simulink model "LRMate200Experimentor_Robot"  (R2015b)
settings: Solver=FixedStepDiscrete  StartTime=0.0  StopTime=10.0  FixedStep=si.SolverTimeStep  RelTol=1e-3
model workspace (MATLAB code in the model file):
  | rsi = evalin('base', 'si.ri{1}');
undefined symbols (not defined in the file or in its folder): si
libraries: simulink x4
(part 1 of 2)
settings Model: xpc_rtwmakecfg_data=_xpcethercatlib_  ParameterArgumentNames=rsi  Creator=rluser  LastModifiedBy=Te Tang
settings SolverCC: EnableConcurrentExecution=on
settings DataIOCC: SaveFormat=Array
settings OptimizationCC: BlockReduction=off  OptimizeBlockIOStorage=off  BufferReuse=off  GlobalBufferReuse=off  ExpressionFolding=off  LocalBlockOutputs=off
settings DebuggingCC: SolverPrmCheckMsg=warning  MultiTaskDSMMsg=none
settings HardwareCC: ProdBitPerPointer=32  ProdLargestAtomicFloat=None  ProdWordSize=32  ProdLongLongMode=on  ProdHWDeviceType=Generic->32-bit x86 compatible
settings RTWCC: SystemTargetFile=slrt.tlc  TemplateMakefile=slrt_default_tmf  Description=Simulink Real-Time  RTWCompilerOptimization=on
settings CodeAppCC: MaxIdLength=120
settings SimulinkRealTimeCC: GeneratePreprocessorConditionals=Disable all
settings ConfigComp: CovModelRefEnable=Off  CovSFcnEnable=off

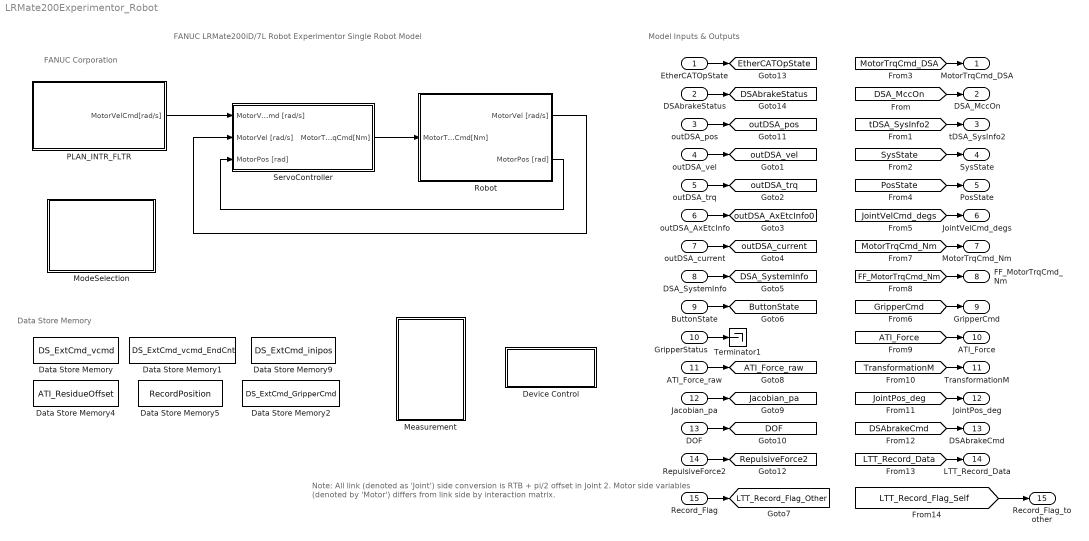
== system LRMate200Experimentor_Robot ==
  note: Model Inputs & Outputs
  note: Data Store Memory
  note: FANUC LRMate200iD/7L Robot Experimentor
      | Single Robot Model
  note: FANUC Corporation
  note: Note: All link (denoted as 'Joint') side conversion is RTB + pi/2 offset in Joint 2.
      | Motor side variables (denoted by 'Motor') differs from link side by interaction matrix.
  EtherCATOpState : Inport
  DSAbrakeStatus : Inport  Port=2
  outDSA_pos : Inport  Port=3
  outDSA_vel : Inport  Port=4
  outDSA_trq : Inport  Port=5
  outDSA_AxEtcInfo : Inport  Port=6
  outDSA_current : Inport  Port=7
  DSA_SystemInfo : Inport  Port=8
  ButtonState : Inport  Port=9  OutDataTypeStr=Bus: ButtonState
  GripperStatus : Inport  Port=10  OutDataTypeStr=Bus: GripperStatus
  ATI_Force_raw : Inport  Port=11  PortDimensions=6
  Jacobian_pa : Inport  Port=12  PortDimensions=[6 6]
  DOF : Inport  Port=13
  RepulsiveForce2 : Inport  Port=14  PortDimensions=3
  Record_Flag : Inport  Port=15  OutDataTypeStr=boolean  PortDimensions=1
  Data Store Memory : DataStoreMemory  DataStoreName=DS_ExtCmd_vcmd  WriteAfterWriteMsg=warning  WriteAfterReadMsg=warning  InitialValue=zeros(si.ext_vel_max_cnt,si.AxisNum)  OutDataTypeStr=double
  Data Store Memory1 : DataStoreMemory  DataStoreName=DS_ExtCmd_vcmd_EndCnt  WriteAfterWriteMsg=warning  WriteAfterReadMsg=warning  OutDataTypeStr=double
  Data Store Memory2 : DataStoreMemory  DataStoreName=DS_ExtCmd_GripperCmd  WriteAfterWriteMsg=warning  WriteAfterReadMsg=warning  InitialValue=zeros(si.ext_vel_max_cnt,6)  OutDataTypeStr=double
  Data Store Memory4 : DataStoreMemory  DataStoreName=ATI_ResidueOffset  WriteAfterWriteMsg=warning  WriteAfterReadMsg=warning  InitialValue=zeros(6,1)  OutDataTypeStr=double
  Data Store Memory5 : DataStoreMemory  DataStoreName=RecordPosition  WriteAfterWriteMsg=warning  WriteAfterReadMsg=warning  InitialValue=zeros(6,1)  OutDataTypeStr=double
  Data Store Memory9 : DataStoreMemory  DataStoreName=DS_ExtCmd_inipos  WriteAfterWriteMsg=warning  WriteAfterReadMsg=warning  InitialValue=zeros(1,si.AxisNum)  VectorParams1D=off  OutDataTypeStr=double
  Device Control : Subsystem
  Measurement : Subsystem
  ModeSelection : Subsystem
  PLAN_INTR_FLTR : Subsystem
  Robot : Subsystem
  ServoController : Subsystem  SystemSampleTime=si.tsv
  Terminator1 : Terminator
  MotorTrqCmd_DSA : Outport
  DSA_MccOn : Outport  Port=2
  tDSA_SysInfo2 : Outport  Port=3
  SysState : Outport  Port=4  OutDataTypeStr=Bus: SysState
  PosState : Outport  Port=5  OutDataTypeStr=Bus: PosState
  JointVelCmd_degs : Outport  Port=6
  MotorTrqCmd_Nm : Outport  Port=7
  FF_MotorTrqCmd_Nm : Outport  Port=8
  GripperCmd : Outport  Port=9  OutDataTypeStr=Bus: GripperCmd
  ATI_Force : Outport  Port=10
  TransformationM : Outport  Port=11
  JointPos_deg : Outport  Port=12
  DSAbrakeCmd : Outport  Port=13
  LTT_Record_Data : Outport  Port=14
  Record_Flag_to other : Outport  Port=15  OutDataTypeStr=boolean  PortDimensions=1
  tag scope: ATI_Force_raw=global, ButtonState=global, DOF=global, DSA_SystemInfo=global, DSAbrakeStatus=global, EtherCATOpState=global, Jacobian_pa=global, LTT_Record_Flag_Other=global, RepulsiveForce2=global, outDSA_AxEtcInfo0=global, outDSA_current=global, outDSA_pos=global, outDSA_trq=global, outDSA_vel=global
  wires:
  PLAN_INTR_FLTR/1(MotorVelCmd[rad/s]) -> ServoController/1(MotorVelCmd [rad/s])
  ServoController/1(MotorTrqCmd[Nm]) -> Robot/1(MotorTrqCmd[Nm])
  Robot/2(MotorPos [rad]) -> ServoController/3(MotorPos [rad])
  Robot/1(MotorVel [rad/s]) -> ServoController/2(MotorVel [rad/s])
  [MotorTrqCmd_DSA] -> MotorTrqCmd_DSA/1
  [DSA_MccOn] -> DSA_MccOn/1
  [tDSA_SysInfo2] -> tDSA_SysInfo2/1
  outDSA_pos/1 -> [outDSA_pos]
  outDSA_vel/1 -> [outDSA_vel]
  outDSA_trq/1 -> [outDSA_trq]
  outDSA_AxEtcInfo/1 -> [outDSA_AxEtcInfo0]
  outDSA_current/1 -> [outDSA_current]
  DSA_SystemInfo/1 -> [DSA_SystemInfo]
  ButtonState/1 -> [ButtonState]
  GripperStatus/1 -> Terminator1/1
  [SysState] -> SysState/1
  [PosState] -> PosState/1
  [JointVelCmd_degs] -> JointVelCmd_degs/1
  [MotorTrqCmd_Nm] -> MotorTrqCmd_Nm/1
  [FF_MotorTrqCmd_Nm] -> FF_MotorTrqCmd_Nm/1
  [GripperCmd] -> GripperCmd/1
  [ATI_Force] -> ATI_Force/1
  [TransformationM] -> TransformationM/1
  ATI_Force_raw/1 -> [ATI_Force_raw]
  [JointPos_deg] -> JointPos_deg/1
  Jacobian_pa/1 -> [Jacobian_pa]
  DOF/1 -> [DOF]
  RepulsiveForce2/1 -> [RepulsiveForce2]
  EtherCATOpState/1 -> [EtherCATOpState]
  DSAbrakeStatus/1 -> [DSAbrakeStatus]
  [DSAbrakeCmd] -> DSAbrakeCmd/1
  [LTT_Record_Data] -> LTT_Record_Data/1
  Record_Flag/1 -> [LTT_Record_Flag_Other]
  [LTT_Record_Flag_Self] -> Record_Flag_to other/1

== system LRMate200Experimentor_Robot/Device Control ==
  Gripper Input : Subsystem
  tag scope: GripperCmd=global
  wires:
  Gripper Input/1(GripperInput) -> [GripperCmd]

== system LRMate200Experimentor_Robot/Measurement ==
  Force Sensor : Subsystem
  LTT Handle : Subsystem
  Position State : Subsystem
  System State : Subsystem
  Terminator1 : Terminator
  Terminator4 : Terminator
  Terminator5 : Terminator
  Tilt Angle Esimation : Subsystem
  tag scope: ATI_Force=global, Green_ButtonE=global, LTT_ButtonE=global, LTT_Force=global, LTT_Record_Data=global, PosState=global, SysState=global, TCP_Force=global
  wires:
  System State/1(System State) -> [SysState]
  Position State/1(Position State) -> [PosState]
  Force Sensor/1(ATI_Force) -> [ATI_Force]
  Force Sensor/2(TCP_Force) -> [TCP_Force]
  LTT Handle/1(Green_Button) -> [Green_ButtonE]
  LTT Handle/2(RecordData) -> [LTT_Record_Data]
  LTT Handle/3(LTT_ButtonEnable) -> [LTT_ButtonE]
  Tilt Angle Esimation/1(Panel_RecordData) -> Terminator5/1
  Tilt Angle Esimation/2(TiltANA_col) -> Terminator4/1
  Tilt Angle Esimation/3(Estimated Tilt Angle) -> Terminator1/1
  Force Sensor/3(LTT_Force) -> [LTT_Force]

== system LRMate200Experimentor_Robot/ModeSelection ==
  Basic Control Mode : Subsystem
  LTT : Subsystem
  Pos Run & Jog : Subsystem

== system LRMate200Experimentor_Robot/PLAN_INTR_FLTR ==
  Basic : Subsystem
  JOG C : Subsystem
  LTT : Subsystem
  Peg Hole Insertion : Subsystem
  MotorVelCmd[rad/s] : Outport
  wires:
  Basic/1(MotorVelCmd[rad/s]) -> MotorVelCmd[rad/s]/1

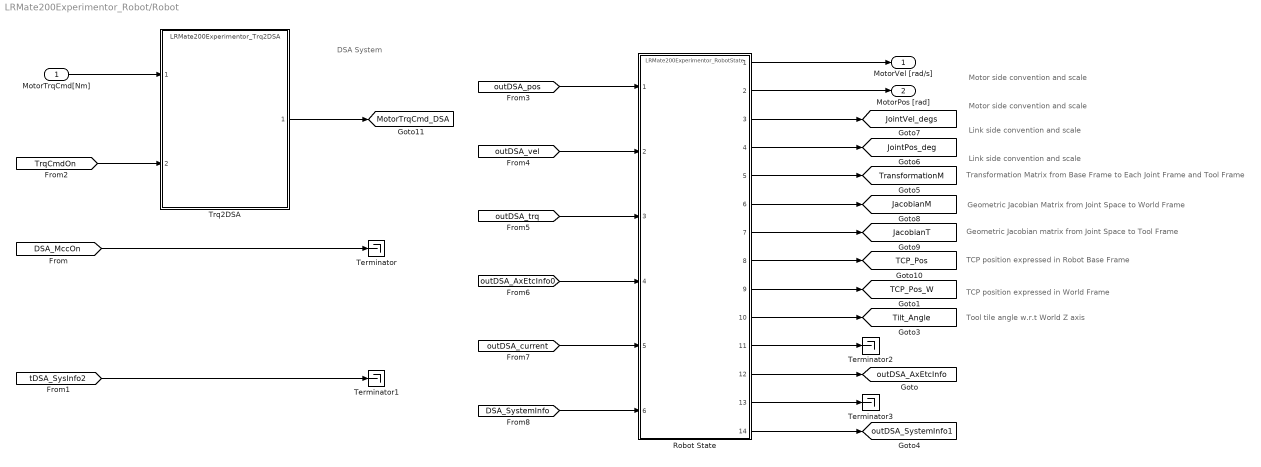
== system LRMate200Experimentor_Robot/Robot ==
  note: Motor side convention and scale
  note: TCP position expressed in Robot Base Frame
  note: Geometric Jacobian matrix from Joint Space to Tool Frame
  note: Geometric Jacobian Matrix from Joint Space to World Frame
  note: Transformation Matrix from Base Frame to Each Joint Frame and Tool Frame
  note: DSA System
  note: Motor side convention and scale
  note: Link side convention and scale
  note: Link side convention and scale
  note: Tool tile angle w.r.t World Z axis
  note: TCP position expressed in World Frame
  MotorTrqCmd[Nm] : Inport
  Robot State : ModelReference  ModelNameDialog=LRMate200Experimentor_RobotState.slx  ParameterArgumentNames=rsi  ParameterArgumentValues=rsi  SimulationMode=Normal  ModelReferenceVersion=1.185  CopyOfModelName=LRMate200Experimentor_RobotState.slx
  Terminator{,1..3} (4 alike) : Terminator
  Trq2DSA : ModelReference  ModelNameDialog=LRMate200Experimentor_Trq2DSA.slx  ParameterArgumentNames=rsi  ParameterArgumentValues=rsi  SimulationMode=Normal  ModelReferenceVersion=1.89  CopyOfModelName=LRMate200Experimentor_Trq2DSA.slx
  MotorVel [rad/s] : Outport
  MotorPos [rad] : Outport  Port=2
  tag scope: JacobianM=global, JacobianT=global, JointPos_deg=global, JointVel_degs=global, MotorTrqCmd_DSA=global, TCP_Pos=global, TCP_Pos_W=global, Tilt_Angle=global, TransformationM=global, outDSA_AxEtcInfo=global, outDSA_SystemInfo1=global
  wires:
  MotorTrqCmd[Nm]/1 -> Trq2DSA/1
  [TrqCmdOn] -> Trq2DSA/2
  [DSA_MccOn] -> Terminator/1
  [tDSA_SysInfo2] -> Terminator1/1
  Robot State/1 -> MotorVel [rad/s]/1
  Robot State/2 -> MotorPos [rad]/1
  Robot State/3 -> [JointVel_degs]
  Robot State/4 -> [JointPos_deg]
  Robot State/5 -> [TransformationM]
  Robot State/6 -> [JacobianM]
  Robot State/7 -> [JacobianT]
  Robot State/8 -> [TCP_Pos]
  Trq2DSA/1 -> [MotorTrqCmd_DSA]
  [outDSA_pos] -> Robot State/1
  [outDSA_vel] -> Robot State/2
  [outDSA_trq] -> Robot State/3
  [outDSA_AxEtcInfo0] -> Robot State/4
  [outDSA_current] -> Robot State/5
  [DSA_SystemInfo] -> Robot State/6
  Robot State/10 -> [Tilt_Angle]
  Robot State/11 -> Terminator2/1
  Robot State/12 -> [outDSA_AxEtcInfo]
  Robot State/13 -> Terminator3/1
  Robot State/14 -> [outDSA_SystemInfo1]
  Robot State/9 -> [TCP_Pos_W]

== system LRMate200Experimentor_Robot/ServoController ==
  MotorVelCmd [rad/s] : Inport
  MotorVel [rad/s] : Inport  Port=2
  MotorPos [rad] : Inport  Port=3
  Servo Model : ModelReference  ModelNameDialog=LRMate200Experimentor_Servo.slx  ParameterArgumentNames=rsi  ParameterArgumentValues=rsi  SimulationMode=Normal  ModelReferenceVersion=1.76  CopyOfModelName=LRMate200Experimentor_Servo.slx
  MotorTrqCmd[Nm] : Outport
  tag scope: FF_MotorTrqCmd_Nm=global, MotorTrqCmd_Nm=global
  wires:
  MotorVelCmd [rad/s]/1 -> Servo Model/1
  MotorPos [rad]/1 -> Servo Model/3
  MotorVel [rad/s]/1 -> Servo Model/2
  [ZReset] -> Servo Model/4
  Servo Model/1 -> [MotorTrqCmd_Nm], MotorTrqCmd[Nm]/1
  Servo Model/2 -> [FF_MotorTrqCmd_Nm]

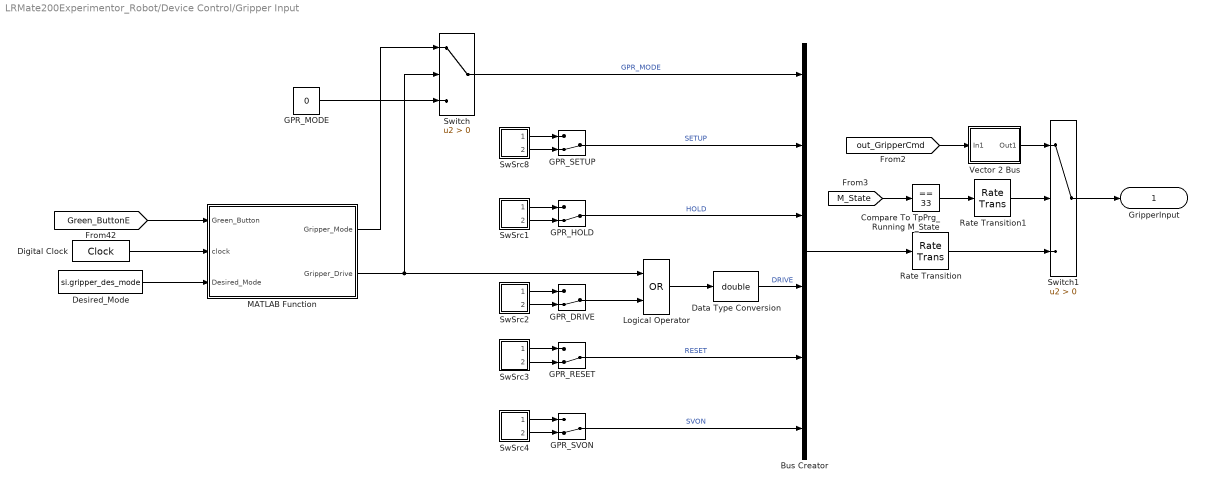
== system LRMate200Experimentor_Robot/Device Control/Gripper Input ==
  Bus Creator : BusCreator  Inputs=6
  Compare To TpPrg_Running M_State : simulink/Logic and Bit Operations/Compare To Constant  relop===  const=33  OutDataTypeStr=boolean
  Data Type Conversion : DataTypeConversion  OutDataTypeStr=double
  Desired_Mode : Constant  Value=si.gripper_des_mode
  Digital Clock : DigitalClock  SampleTime=0.001
  GPR_DRIVE : ManualSwitch  CurrentSetting=0
  GPR_HOLD : ManualSwitch  CurrentSetting=0
  GPR_MODE : Constant  Value=0
  GPR_RESET : ManualSwitch  CurrentSetting=0
  GPR_SETUP : ManualSwitch  CurrentSetting=0
  GPR_SVON : ManualSwitch  CurrentSetting=0
  Logical Operator : Logic  Operator=OR  AllPortsSameDT=off  OutDataTypeStr=boolean
  MATLAB Function : MATLAB Function  TreatAsAtomicUnit=on
  Rate Transition : RateTransition  OutPortSampleTime=si.timeGripperInputHold
  Rate Transition1 : RateTransition  OutPortSampleTime=si.timeGripperInputHold
  SwSrc1 : Subsystem
  SwSrc2 : Subsystem
  SwSrc3 : Subsystem
  SwSrc4 : Subsystem
  SwSrc8 : Subsystem
  Switch : Switch  Criteria=u2 > Threshold
  Switch1 : Switch  Criteria=u2 > Threshold
  Vector 2 Bus : Subsystem
  GripperInput : Outport
  wires:
  GPR_SVON/1 -> Bus Creator/6  "SVON"
  SwSrc8/2(ST0) -> GPR_SETUP/2
  SwSrc1/2(ST0) -> GPR_HOLD/2
  SwSrc4/2(ST0) -> GPR_SVON/2
  SwSrc1/1(ST1) -> GPR_HOLD/1
  SwSrc8/1(ST1) -> GPR_SETUP/1
  GPR_HOLD/1 -> Bus Creator/3  "HOLD"
  GPR_SETUP/1 -> Bus Creator/2  "SETUP"
  GPR_RESET/1 -> Bus Creator/5  "RESET"
  SwSrc2/2(ST0) -> GPR_DRIVE/2
  SwSrc3/2(ST0) -> GPR_RESET/2
  SwSrc4/1(ST1) -> GPR_SVON/1
  SwSrc3/1(ST1) -> GPR_RESET/1
  SwSrc2/1(ST1) -> GPR_DRIVE/1
  Digital Clock/1 -> MATLAB Function/2(clock)
  [Green_ButtonE] -> MATLAB Function/1(Green_Button)
  Logical Operator/1 -> Data Type Conversion/1
  GPR_DRIVE/1 -> Logical Operator/2
  MATLAB Function/2(Gripper_Drive) -> Switch/2, Logical Operator/1
  Switch/1 -> Bus Creator/1  "GPR_MODE"
  GPR_MODE/1 -> Switch/3
  MATLAB Function/1(Gripper_Mode) -> Switch/1
  Data Type Conversion/1 -> Bus Creator/4  "DRIVE"
  [out_GripperCmd] -> Vector 2 Bus/1(In1)
  Compare To TpPrg_Running M_State/1 -> Rate Transition1/1
  Bus Creator/1 -> Rate Transition/1
  Vector 2 Bus/1(Out1) -> Switch1/1
  Switch1/1 -> GripperInput/1
  Rate Transition/1 -> Switch1/3
  Rate Transition1/1 -> Switch1/2
  [M_State] -> Compare To TpPrg_Running M_State/1
  Desired_Mode/1 -> MATLAB Function/3(Desired_Mode)

== system LRMate200Experimentor_Robot/Measurement/Force Sensor ==
  ATI_Offset : Constant  Value=rsi.ATI_Offset
  Calibratioin Matrix : Gain  Gain=rsi.CalibrationMatrix  Multiplication=Matrix(K*u) (u vector)
  Data Store Read : DataStoreRead  DialogController=Simulink.DDGSource  DataStoreName=ATI_ResidueOffset  SampleTime=si.tsv
  Discrete Filter : DiscreteFilter  Numerator=si.Filter.num  Denominator=si.Filter.den  SampleTime=si.tsv
  Discrete Filter1 : DiscreteFilter  Numerator=si.Filter.num  Denominator=si.Filter.den  SampleTime=si.tsv
  Gravity Compensator : MATLAB Function  TreatAsAtomicUnit=on
  L_ATI2LTT : Constant  Value=rsi.L_ATI2LTT
  L_ATI2TCP : Constant  Value=rsi.L_ATI2TCP
  MATLAB Function6 : MATLAB Function  TreatAsAtomicUnit=on
  PayloadCG : Constant  Value=rsi.PayloadCG
  PayloadG : Constant  Value=rsi.PayloadG
  Substract : Sum  Inputs=+---
  ATI_Force : Outport
  TCP_Force : Outport  Port=2
  LTT_Force : Outport  Port=3
  wires:
  PayloadCG/1 -> Gravity Compensator/3(PayloadCG)
  [ATI_Force_raw] -> Calibratioin Matrix/1
  [TransformationM] -> Gravity Compensator/1(T)
  PayloadG/1 -> Gravity Compensator/2(PayloadG)
  Gravity Compensator/1(W) -> Discrete Filter1/1
  ATI_Offset/1 -> Substract/2
  Discrete Filter1/1 -> Substract/3
  Substract/1 -> ATI_Force/1, MATLAB Function6/1(ATI_Force)
  Calibratioin Matrix/1 -> Discrete Filter/1
  Discrete Filter/1 -> Substract/1
  Data Store Read/1 -> Substract/4
  MATLAB Function6/1(TCP_Force) -> TCP_Force/1
  L_ATI2TCP/1 -> MATLAB Function6/2(L_ATI2TCP)
  L_ATI2LTT/1 -> MATLAB Function6/3(L_ATI2LTT)
  MATLAB Function6/2(LTT_Force) -> LTT_Force/1

== system LRMate200Experimentor_Robot/Measurement/LTT Handle ==
  Bus Selector : BusSelector  OutputSignals=Green_Button,LTT_Button
  Digital Clock : DigitalClock  SampleTime=0.001
  LTT_RecordData_On : Constant  Value=0
  MATLAB Function : MATLAB Function  TreatAsAtomicUnit=on
  Mux : Mux  Inputs=3
  Rate Transition : RateTransition
  Rate Transition1 : RateTransition
  Green_Button : Outport
  RecordData : Outport  Port=2
  LTT_ButtonEnable : Outport  Port=3
  tag scope: LTT_Record_Flag_Self=global
  wires:
  MATLAB Function/1(RecordData) -> RecordData/1
  Digital Clock/1 -> MATLAB Function/4(clock)
  MATLAB Function/2(LTT_ButtonEnable) -> LTT_ButtonEnable/1
  Mux/1 -> MATLAB Function/3(DATA)
  [JointPos_deg] -> Mux/1
  Bus Selector/2 -> MATLAB Function/1(LTT_Button)  "<LTT_Button>"
  Bus Selector/1 -> Green_Button/1  "<Green_Button>"
  [ButtonState] -> Bus Selector/1
  [LTTCmd_E] -> Rate Transition1/1
  Rate Transition1/1 -> MATLAB Function/2(LTTCmd_E)
  [LTT_Force] -> Mux/3
  [GripperCmd] -> Rate Transition/1
  Rate Transition/1 -> Mux/2
  LTT_RecordData_On/1 -> MATLAB Function/5(RecordDataOn)
  [LTT_Record_Flag_Other] -> MATLAB Function/6(Record_Flag_Other)
  MATLAB Function/3(Record_Flag_Self) -> [LTT_Record_Flag_Self]

== system LRMate200Experimentor_Robot/Measurement/Position State ==
  Bus Creator1 : BusCreator  Inputs=9
  Demux1 : Demux  Outputs=6
  Demux2 : Demux  Outputs=3
  Gain{5,14..18} (6 alike) : Gain
  Gain2 : Gain  Gain=1000
  Gain3 : Gain  Gain=1000
  Gain4 : Gain  Gain=1000
  Position State : Outport
  wires:
  [JointPos_deg] -> Demux1/1
  Demux1/1 -> Gain5/1
  Demux1/2 -> Gain14/1
  Demux1/3 -> Gain15/1
  Demux1/6 -> Gain18/1
  Demux1/5 -> Gain17/1
  Demux1/4 -> Gain16/1
  Gain18/1 -> Bus Creator1/6  "Pos_J6_deg"
  Gain17/1 -> Bus Creator1/5  "Pos_J5_deg"
  Gain16/1 -> Bus Creator1/4  "Pos_J4_deg"
  Gain15/1 -> Bus Creator1/3  "Pos_J3_deg"
  Gain14/1 -> Bus Creator1/2  "Pos_J2_deg"
  Gain5/1 -> Bus Creator1/1  "Pos_J1_deg"
  Bus Creator1/1 -> Position State/1
  [TCP_Pos] -> Demux2/1
  Demux2/1 -> Gain2/1
  Demux2/2 -> Gain3/1
  Demux2/3 -> Gain4/1
  Gain2/1 -> Bus Creator1/7  "Pos_X_mm"
  Gain3/1 -> Bus Creator1/8  "Pos_Y_mm"
  Gain4/1 -> Bus Creator1/9  "Pos_Z_mm"

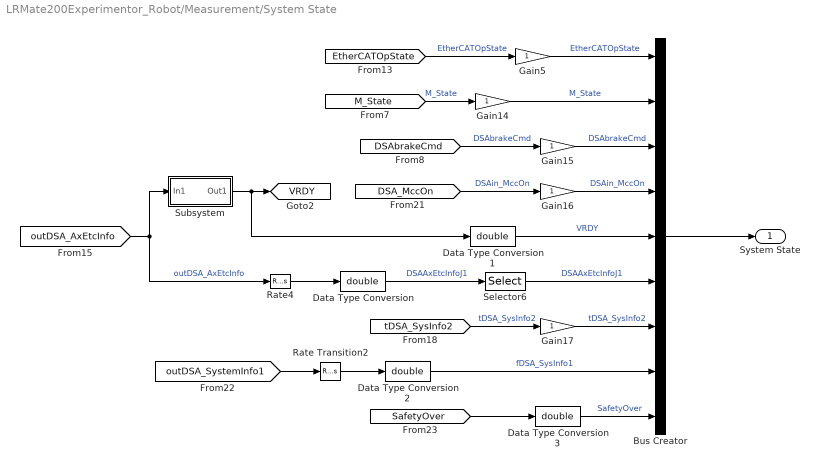
== system LRMate200Experimentor_Robot/Measurement/System State ==
  Bus Creator : BusCreator  Inputs=9
  Data Type Conversion{,1..3} (4 alike) : DataTypeConversion  OutDataTypeStr=double
  Gain{5,14..17} (5 alike) : Gain
  Rate Transition2 : RateTransition
  Rate4 : RateTransition
  Selector6 : Selector  InputPortWidth=6  IndexOptions=Index vector (dialog)  Indices=[1]  OutputSizes=1
  Subsystem : Subsystem
  System State : Outport
  tag scope: VRDY=global
  wires:
  [M_State] -> Gain14/1  "M_State"
  [DSAbrakeCmd] -> Gain15/1  "DSAbrakeCmd"
  [EtherCATOpState] -> Gain5/1  "EtherCATOpState"
  Bus Creator/1 -> System State/1
  [outDSA_AxEtcInfo] -> Rate4/1, Subsystem/1(In1)  "outDSA_AxEtcInfo"
  [DSA_MccOn] -> Gain16/1  "DSAin_MccOn"
  Rate4/1 -> Data Type Conversion/1
  Data Type Conversion/1 -> Selector6/1  "DSAAxEtcInfoJ1"
  Selector6/1 -> Bus Creator/6  "DSAAxEtcInfoJ1"
  Subsystem/1(Out1) -> Data Type Conversion1/1, [VRDY]
  Data Type Conversion1/1 -> Bus Creator/5  "VRDY"
  [tDSA_SysInfo2] -> Gain17/1  "tDSA_SysInfo2"
  [outDSA_SystemInfo1] -> Rate Transition2/1
  Rate Transition2/1 -> Data Type Conversion2/1
  Data Type Conversion2/1 -> Bus Creator/8  "fDSA_SysInfo1"
  [SafetyOver] -> Data Type Conversion3/1
  Data Type Conversion3/1 -> Bus Creator/9  "SafetyOver"
  Gain15/1 -> Bus Creator/3  "DSAbrakeCmd"
  Gain16/1 -> Bus Creator/4  "DSAin_MccOn"
  Gain14/1 -> Bus Creator/2  "M_State"
  Gain5/1 -> Bus Creator/1  "EtherCATOpState"
  Gain17/1 -> Bus Creator/7  "tDSA_SysInfo2"

== system LRMate200Experimentor_Robot/Measurement/Tilt Angle Esimation ==
  MATLAB Function2 : MATLAB Function  TreatAsAtomicUnit=on
  Mux2 : Mux  Inputs=5
  PanelREC : Constant  Value=0
  TiltEstimate : MATLAB Function  TreatAsAtomicUnit=on
  Panel_RecordData : Outport
  TiltANA_col : Outport  Port=2
  Estimated Tilt Angle : Outport  Port=3
  wires:
  TiltEstimate/1(TiltANA_col) -> TiltANA_col/1
  TiltEstimate/2(Alpha) -> Estimated Tilt Angle/1
  [TCP_Force] -> TiltEstimate/1(TCP_Force)
  [TransformationM] -> TiltEstimate/2(TransformationM)
  [JointPos_deg] -> TiltEstimate/3(JointPos_deg)
  Mux2/1 -> MATLAB Function2/2(DATA)
  [JointPos_deg] -> Mux2/1
  [TCP_Pos] -> Mux2/2
  MATLAB Function2/1(RecordData) -> Panel_RecordData/1
  PanelREC/1 -> MATLAB Function2/1(Button)
  [TCP_Force] -> Mux2/4
  [Tilt_Angle] -> Mux2/5
  [ATI_Force] -> Mux2/3

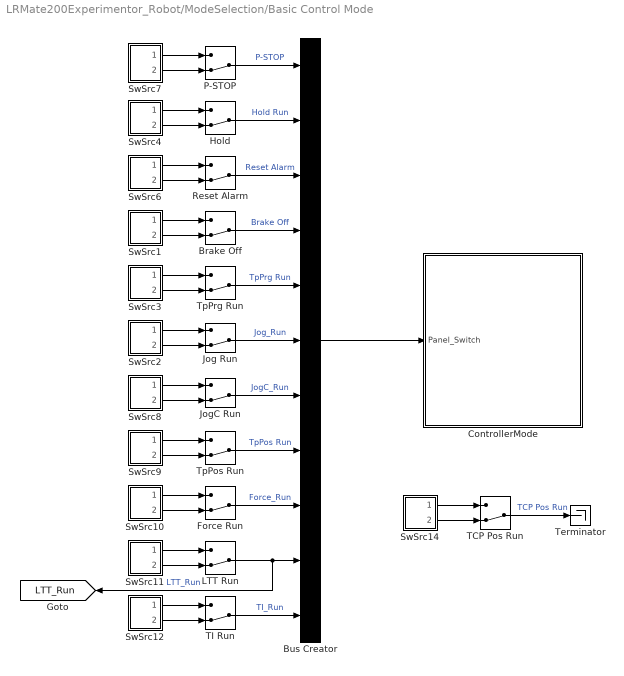
== system LRMate200Experimentor_Robot/ModeSelection/Basic Control Mode ==
  Brake Off : ManualSwitch  CurrentSetting=0
  Bus Creator : BusCreator  Inputs=11
  ControllerMode : Subsystem
  Force Run : ManualSwitch  CurrentSetting=0
  Hold : ManualSwitch  CurrentSetting=0
  Jog Run : ManualSwitch  CurrentSetting=0
  JogC Run : ManualSwitch  CurrentSetting=0
  LTT Run : ManualSwitch  CurrentSetting=0
  P-STOP : ManualSwitch  CurrentSetting=0
  Reset Alarm : ManualSwitch  CurrentSetting=0
  SwSrc1 : Subsystem
  SwSrc10 : Subsystem
  SwSrc11 : Subsystem
  SwSrc12 : Subsystem
  SwSrc14 : Subsystem
  SwSrc2 : Subsystem
  SwSrc3 : Subsystem
  SwSrc4 : Subsystem
  SwSrc6 : Subsystem
  SwSrc7 : Subsystem
  SwSrc8 : Subsystem
  SwSrc9 : Subsystem
  TCP Pos Run : ManualSwitch  CurrentSetting=0
  TI Run : ManualSwitch  CurrentSetting=0
  Terminator : Terminator
  TpPos Run : ManualSwitch  CurrentSetting=0
  TpPrg Run : ManualSwitch  CurrentSetting=0
  tag scope: LTT_Run=global
  wires:
  SwSrc9/1(ST1) -> TpPos Run/1
  TpPos Run/1 -> Bus Creator/8  "TpPos Run"
  SwSrc9/2(ST0) -> TpPos Run/2
  Brake Off/1 -> Bus Creator/4  "Brake Off"
  Jog Run/1 -> Bus Creator/6  "Jog_Run"
  TpPrg Run/1 -> Bus Creator/5  "TpPrg Run"
  Hold/1 -> Bus Creator/2  "Hold Run"
  SwSrc1/1(ST1) -> Brake Off/1
  SwSrc2/1(ST1) -> Jog Run/1
  SwSrc2/2(ST0) -> Jog Run/2
  SwSrc3/1(ST1) -> TpPrg Run/1
  SwSrc3/2(ST0) -> TpPrg Run/2
  SwSrc4/2(ST0) -> Hold/2
  Bus Creator/1 -> ControllerMode/1(Panel_Switch)
  SwSrc6/1(ST1) -> Reset Alarm/1
  SwSrc6/2(ST0) -> Reset Alarm/2
  Reset Alarm/1 -> Bus Creator/3  "Reset Alarm"
  SwSrc7/1(ST1) -> P-STOP/1
  SwSrc7/2(ST0) -> P-STOP/2
  P-STOP/1 -> Bus Creator/1  "P-STOP"
  SwSrc4/1(ST1) -> Hold/1
  JogC Run/1 -> Bus Creator/7  "JogC_Run"
  SwSrc8/1(ST1) -> JogC Run/1
  SwSrc8/2(ST0) -> JogC Run/2
  SwSrc1/2(ST0) -> Brake Off/2
  SwSrc10/1(ST1) -> Force Run/1
  Force Run/1 -> Bus Creator/9  "Force_Run"
  SwSrc10/2(ST0) -> Force Run/2
  SwSrc11/1(ST1) -> LTT Run/1
  LTT Run/1 -> [LTT_Run], Bus Creator/10  "LTT_Run"
  SwSrc11/2(ST0) -> LTT Run/2
  SwSrc12/1(ST1) -> TI Run/1
  TI Run/1 -> Bus Creator/11  "TI_Run"
  SwSrc12/2(ST0) -> TI Run/2
  SwSrc14/1(ST1) -> TCP Pos Run/1
  TCP Pos Run/1 -> Terminator/1  "TCP Pos Run"
  SwSrc14/2(ST0) -> TCP Pos Run/2

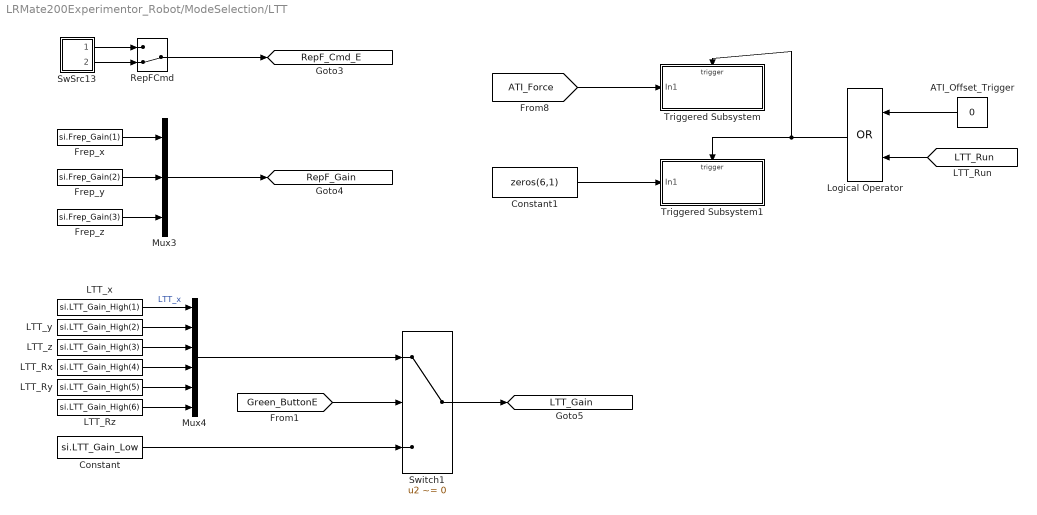
== system LRMate200Experimentor_Robot/ModeSelection/LTT ==
  ATI_Offset_Trigger : Constant  Value=0  OutDataTypeStr=boolean
  Constant : Constant  Value=si.LTT_Gain_Low
  Constant1 : Constant  Value=zeros(6,1)
  Frep_x : Constant  Value=si.Frep_Gain(1)
  Frep_y : Constant  Value=si.Frep_Gain(2)
  Frep_z : Constant  Value=si.Frep_Gain(3)
  LTT_Rx : Constant  Value=si.LTT_Gain_High(4)
  LTT_Ry : Constant  Value=si.LTT_Gain_High(5)
  LTT_Rz : Constant  Value=si.LTT_Gain_High(6)
  LTT_x : Constant  Value=si.LTT_Gain_High(1)
  LTT_y : Constant  Value=si.LTT_Gain_High(2)
  LTT_z : Constant  Value=si.LTT_Gain_High(3)
  Logical Operator : Logic  Operator=OR  AllPortsSameDT=off  OutDataTypeStr=boolean
  Mux3 : Mux  Inputs=3
  Mux4 : Mux  Inputs=6
  RepFCmd : ManualSwitch  CurrentSetting=0
  SwSrc13 : Subsystem
  Switch1 : Switch  Criteria=u2 ~= 0
  Triggered Subsystem : Subsystem  TreatAsAtomicUnit=on
  Triggered Subsystem1 : Subsystem  TreatAsAtomicUnit=on
  tag scope: LTT_Gain=global, RepF_Cmd_E=global, RepF_Gain=global
  wires:
  SwSrc13/1(ST1) -> RepFCmd/1
  SwSrc13/2(ST0) -> RepFCmd/2
  RepFCmd/1 -> [RepF_Cmd_E]
  Frep_x/1 -> Mux3/1
  Frep_z/1 -> Mux3/3
  Frep_y/1 -> Mux3/2
  Mux3/1 -> [RepF_Gain]
  LTT_x/1 -> Mux4/1  "LTT_x"
  LTT_z/1 -> Mux4/3
  LTT_y/1 -> Mux4/2
  Mux4/1 -> Switch1/1
  Switch1/1 -> [LTT_Gain]
  [Green_ButtonE] -> Switch1/2
  LTT_Ry/1 -> Mux4/5
  LTT_Rz/1 -> Mux4/6
  LTT_Rx/1 -> Mux4/4
  Constant/1 -> Switch1/3
  Logical Operator/1 -> Triggered Subsystem/Trigger, Triggered Subsystem1/Trigger
  Constant1/1 -> Triggered Subsystem1/1(In1)
  [ATI_Force] -> Triggered Subsystem/1(In1)
  ATI_Offset_Trigger/1 -> Logical Operator/1
  [LTT_Run] -> Logical Operator/2

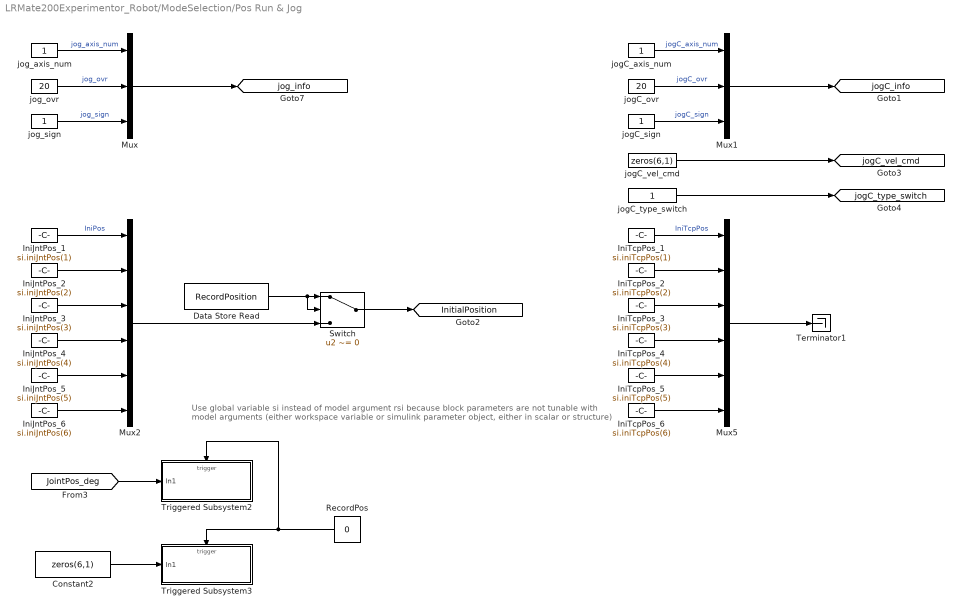
== system LRMate200Experimentor_Robot/ModeSelection/Pos Run & Jog ==
  note: Use global variable si instead of model argument rsi because block parameters are not tunable
      | with model arguments (either workspace variable or simulink parameter object, either in scalar or structure)
  Constant2 : Constant  Value=zeros(6,1)
  Data Store Read : DataStoreRead  DialogController=Simulink.DDGSource  DataStoreName=RecordPosition  SampleTime=si.itp
  IniJntPos_1 : Constant  Value=si.iniJntPos(1)
  IniJntPos_2 : Constant  Value=si.iniJntPos(2)
  IniJntPos_3 : Constant  Value=si.iniJntPos(3)
  IniJntPos_4 : Constant  Value=si.iniJntPos(4)
  IniJntPos_5 : Constant  Value=si.iniJntPos(5)
  IniJntPos_6 : Constant  Value=si.iniJntPos(6)
  IniTcpPos_1 : Constant  Value=si.iniTcpPos(1)
  IniTcpPos_2 : Constant  Value=si.iniTcpPos(2)
  IniTcpPos_3 : Constant  Value=si.iniTcpPos(3)
  IniTcpPos_4 : Constant  Value=si.iniTcpPos(4)
  IniTcpPos_5 : Constant  Value=si.iniTcpPos(5)
  IniTcpPos_6 : Constant  Value=si.iniTcpPos(6)
  Mux : Mux  Inputs=3
  Mux1 : Mux  Inputs=3
  Mux2 : Mux  Inputs=6
  Mux5 : Mux  Inputs=6
  RecordPos : Constant  Value=0  OutDataTypeStr=boolean
  Switch : Switch  Criteria=u2 ~= 0
  Terminator1 : Terminator
  Triggered Subsystem2 : Subsystem  TreatAsAtomicUnit=on
  Triggered Subsystem3 : Subsystem  TreatAsAtomicUnit=on
  jogC_axis_num : Constant
  jogC_ovr : Constant  Value=20
  jogC_sign : Constant
  jogC_type_switch : Constant
  jogC_vel_cmd : Constant  Value=zeros(6,1)
  jog_axis_num : Constant
  jog_ovr : Constant  Value=20
  jog_sign : Constant
  tag scope: InitialPosition=global, jogC_info=global, jogC_type_switch=global, jogC_vel_cmd=global, jog_info=global
  wires:
  jog_axis_num/1 -> Mux/1  "jog_axis_num"
  jog_ovr/1 -> Mux/2  "jog_ovr"
  jog_sign/1 -> Mux/3  "jog_sign"
  Mux/1 -> [jog_info]
  jogC_axis_num/1 -> Mux1/1  "jogC_axis_num"
  jogC_ovr/1 -> Mux1/2  "jogC_ovr"
  jogC_sign/1 -> Mux1/3  "jogC_sign"
  Mux1/1 -> [jogC_info]
  IniJntPos_1/1 -> Mux2/1  "IniPos"
  IniJntPos_4/1 -> Mux2/4
  IniJntPos_5/1 -> Mux2/5
  IniJntPos_3/1 -> Mux2/3
  IniJntPos_6/1 -> Mux2/6
  IniJntPos_2/1 -> Mux2/2
  RecordPos/1 -> Triggered Subsystem2/Trigger, Triggered Subsystem3/Trigger
  Constant2/1 -> Triggered Subsystem3/1(In1)
  [JointPos_deg] -> Triggered Subsystem2/1(In1)
  Mux2/1 -> Switch/3
  Switch/1 -> [InitialPosition]
  Data Store Read/1 -> Switch/2, Switch/1
  IniTcpPos_1/1 -> Mux5/1  "IniTcpPos"
  IniTcpPos_4/1 -> Mux5/4
  IniTcpPos_5/1 -> Mux5/5
  IniTcpPos_3/1 -> Mux5/3
  IniTcpPos_6/1 -> Mux5/6
  IniTcpPos_2/1 -> Mux5/2
  Mux5/1 -> Terminator1/1
  jogC_vel_cmd/1 -> [jogC_vel_cmd]
  jogC_type_switch/1 -> [jogC_type_switch]

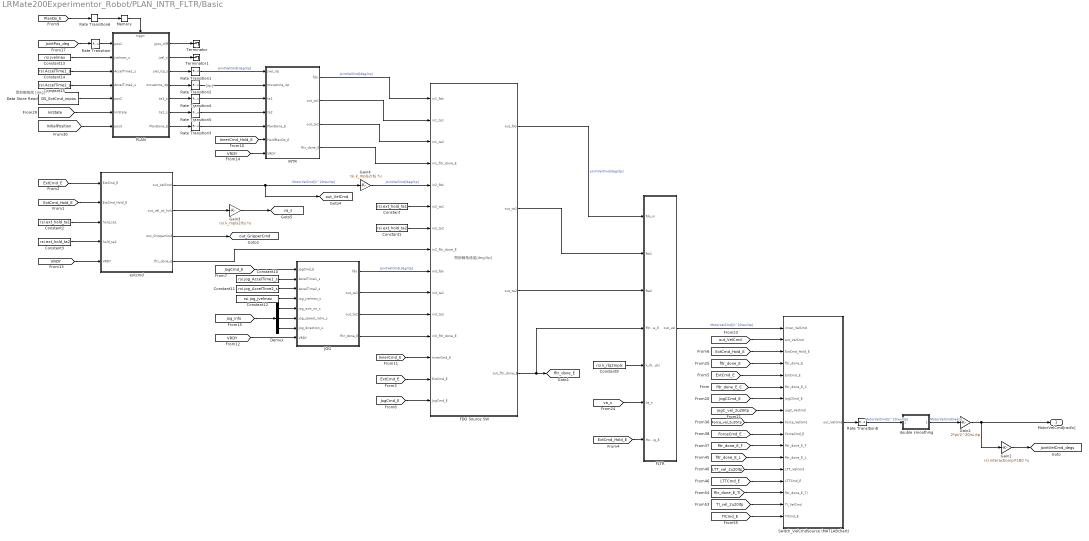
== system LRMate200Experimentor_Robot/PLAN_INTR_FLTR/Basic ==
  note: [itp]
  note: 関節軸角度
      | [deg]
  note: 関節軸角速度[deg/itp]
  Constant : Constant  Value=rsi.ext_hold_ta1  SampleTime=si.itp
  Constant1 : Constant  Value=rsi.ext_hold_ta2  SampleTime=si.itp
  Constant10 : Constant  Value=rsi.jog_AccelTime1_s  SampleTime=si.itp
  Constant11 : Constant  Value=rsi.jog_AccelTime2_s  SampleTime=si.itp
  Constant12 : Constant  Value=rsi.jog_jvelmax  SampleTime=si.itp
  Constant13 : Constant  Value=rsi.jvelmax  SampleTime=si.itp
  Constant14 : Constant  Value=rsi.AccelTime1_s  SampleTime=si.itp
  Constant15 : Constant  Value=rsi.AccelTime2_s  SampleTime=si.itp
  Constant2 : Constant  Value=rsi.ext_hold_ta1  SampleTime=si.itp
  Constant3 : Constant  Value=rsi.ext_hold_ta2  SampleTime=si.itp
  Constant9 : Constant  Value=rsi.k_rbj2mpls  SampleTime=si.itp
  Data Store Read : DataStoreRead  DialogController=Simulink.DDGSource  DataStoreName=DS_ExtCmd_inipos  SampleTime=si.itp
  Demux : Demux  Outputs=3
  FDO Source SW : Stateflow chart  TreatAsAtomicUnit=on
  FLTR : Stateflow chart  TreatAsAtomicUnit=on
  Gain1 : Gain  Gain=rsi.interaction/pi*180  Multiplication=Matrix(K*u)
  Gain2 : Gain  Gain=2*pi/2^20/si.itp
  Gain3 : Gain  Gain=rsi.k_mpls2rbj  Multiplication=Matrix(K*u) (u vector)
  Gain4 : Gain  Gain=rsi.k_mpls2rbj  Multiplication=Matrix(K*u) (u vector)
  INTR : Stateflow chart  TreatAsAtomicUnit=on
  JOG : Stateflow chart  TreatAsAtomicUnit=on
  Memory : Memory  InheritSampleTime=on
  PLAN : Stateflow chart  TreatAsAtomicUnit=on
  Rate Transition{,1..6,8} (8 alike) : RateTransition
  Switch_VelCmdSource (MATLABchart) : Stateflow chart  TreatAsAtomicUnit=on
  Terminator : Terminator
  Terminator1 : Terminator
  double smoothing : Subsystem
  extcmd : Stateflow chart  TreatAsAtomicUnit=on
  MotorVelCmd[rad/s] : Outport
  tag scope: JointVelCmd_degs=global, fltr_done_E=global, out_GripperCmd=global, out_VelCmd=global, va_s=global
  wires:
  PLAN/3(jvel_itp_s) -> Rate Transition1/1
  PLAN/4(movetime_itp) -> Rate Transition2/1
  PLAN/7(PlanDone_E) -> Rate Transition3/1
  INTR/1(fdo) -> FDO Source SW/1(in1_fdo)  "JointVelCmd[deg/itp]"
  PLAN/1(jpos_diff) -> Terminator/1
  PLAN/5(ta1_s) -> Rate Transition4/1
  PLAN/6(ta2_s) -> Rate Transition5/1
  INTR/2(out_ta1) -> FDO Source SW/2(in1_ta1)
  INTR/3(out_ta2) -> FDO Source SW/3(in1_ta2)
  INTR/4(fltr_done_E) -> FDO Source SW/4(in1_fltr_done_E)
  Rate Transition/1 -> PLAN/1(pos1)
  [PlanDo_E] -> Rate Transition6/1
  Rate Transition1/1 -> INTR/1(jvel_itp)  "JointVelCmd[deg/itp]"
  Rate Transition2/1 -> INTR/2(movetime_itp)
  Rate Transition3/1 -> INTR/5(PlanDone_E)
  Rate Transition4/1 -> INTR/3(ta1)
  Rate Transition5/1 -> INTR/4(ta2)
  Rate Transition6/1 -> Memory/1
  Memory/1 -> PLAN/Trigger
  FLTR/1(out_vel) -> Switch_VelCmdSource (MATLABchart)/1(inner_VelCmd)  "MotorVelCmd[2^20rev/itp]"
  [JointPos_deg] -> Rate Transition/1
  FDO Source SW/1(out_fdo) -> FLTR/1(fdo_in)  "JointVelCmd[deg/itp]"
  FDO Source SW/2(out_ta1) -> FLTR/2(fta1)
  FDO Source SW/3(out_ta2) -> FLTR/3(fta2)
  [ExtCmd_E] -> extcmd/1(ExtCmd_E)
  Constant/1 -> FDO Source SW/6(in2_ta1)
  Constant1/1 -> FDO Source SW/7(in2_ta2)
  extcmd/4(fltr_done_E) -> FDO Source SW/8(in2_fltr_done_E)
  [ExtCmd_Hold_E] -> extcmd/2(ExtCmd_Hold_E)
  [ExtCmd_Hold_E] -> Switch_VelCmdSource (MATLABchart)/3(ExtCmd_Hold_E)
  FDO Source SW/4(out_fltr_done_E) -> [fltr_done_E], FLTR/4(fltr_done_E)
  extcmd/2(out_vel_at_hold) -> Gain3/1
  Constant2/1 -> extcmd/3(hold_ta1)
  Constant3/1 -> extcmd/4(hold_ta2)
  extcmd/1(out_VelCmd) -> [out_VelCmd], Gain4/1  "MotorVelCmd[2^20rev/itp]"
  Gain4/1 -> FDO Source SW/5(in2_fdo)  "JointVelCmd[deg/itp]"
  [ExtCmd_Hold_E] -> FLTR/7(HoldSig_E)
  [ExtCmd_E] -> Switch_VelCmdSource (MATLABchart)/5(ExtCmd_E)
  [InnerCmd_E] -> FDO Source SW/13(InnerCmd_E)
  [ExtCmd_E] -> FDO Source SW/14(ExtCmd_E)
  Data Store Read/1 -> PLAN/5(pos2)
  JOG/1(fdo) -> FDO Source SW/9(in3_fdo)  "JointVelCmd[deg/itp]"
  JOG/2(out_ta1) -> FDO Source SW/10(in3_ta1)
  JOG/3(out_ta2) -> FDO Source SW/11(in3_ta2)
  JOG/4(fltr_done_E) -> FDO Source SW/12(in3_fltr_done_E)
  [JogCmd_E] -> JOG/1(JogCmd_E)
  [JogCmd_E] -> FDO Source SW/15(JogCmd_E)
  PLAN/2(jvel_s) -> Terminator1/1
  [VRDY] -> JOG/8(VRDY)
  [VRDY] -> extcmd/5(VRDY)
  [VRDY] -> INTR/7(VRDY)
  [jog_info] -> Demux/1
  Demux/1 -> JOG/5(jog_axis_no_s)
  Demux/2 -> JOG/6(jog_speed_ratio_s)
  Demux/3 -> JOG/7(jog_direction_s)
  [InnerCmd_Hold_E] -> INTR/6(HoldPlanDo_E)
  [fltr_done_E_C] -> Switch_VelCmdSource (MATLABchart)/6(fltr_done_E_C)
  [JogCCmd_E] -> Switch_VelCmdSource (MATLABchart)/7(JogCCmd_E)
  [jogC_vel_2u20itp] -> Switch_VelCmdSource (MATLABchart)/8(jogC_VelCmd)
  [out_VelCmd] -> Switch_VelCmdSource (MATLABchart)/2(ext_VelCmd)
  Gain3/1 -> [va_s]
  [va_s] -> FLTR/6(va_s)
  [fltr_done_E] -> Switch_VelCmdSource (MATLABchart)/4(fltr_done_E)
  [IniState] -> PLAN/6(IniState)
  [InitialPosition] -> PLAN/7(pos3)
  Switch_VelCmdSource (MATLABchart)/1(out_VelCmd) -> Rate Transition8/1
  [Force_vel_2u20itp] -> Switch_VelCmdSource (MATLABchart)/9(Force_VelCmd)
  [ForceCmd_E] -> Switch_VelCmdSource (MATLABchart)/10(ForceCmd_E)
  [fltr_done_E_F] -> Switch_VelCmdSource (MATLABchart)/11(fltr_done_E_F)
  Gain1/1 -> [JointVelCmd_degs]
  [fltr_done_E_L] -> Switch_VelCmdSource (MATLABchart)/12(fltr_done_E_L)
  Rate Transition8/1 -> double smoothing/1(mcmd)  "MotorVelCmd[2^20rev/itp]"
  double smoothing/1(alt_efot) -> Gain2/1  "MotorVelCmd[rad/s]"
  Gain2/1 -> MotorVelCmd[rad/s]/1, Gain1/1
  [LTT_vel_2u20itp] -> Switch_VelCmdSource (MATLABchart)/13(LTT_VelCmd)
  [LTTCmd_E] -> Switch_VelCmdSource (MATLABchart)/14(LTTCmd_E)
  [fltr_done_E_TI] -> Switch_VelCmdSource (MATLABchart)/15(fltr_done_E_TI)
  [TI_vel_2u20itp] -> Switch_VelCmdSource (MATLABchart)/16(TI_VelCmd)
  [TICmd_E] -> Switch_VelCmdSource (MATLABchart)/17(TICmd_E)
  Constant9/1 -> FLTR/5(k_rbj2mpls)
  Constant10/1 -> JOG/2(AccelTime1_s)
  Constant11/1 -> JOG/3(AccelTime2_s)
  Constant12/1 -> JOG/4(jog_jvelmax_s)
  Constant13/1 -> PLAN/2(jvelmax_s)
  Constant14/1 -> PLAN/3(AccelTime1_s)
  Constant15/1 -> PLAN/4(AccelTime2_s)
  extcmd/3(out_GripperCmd) -> [out_GripperCmd]

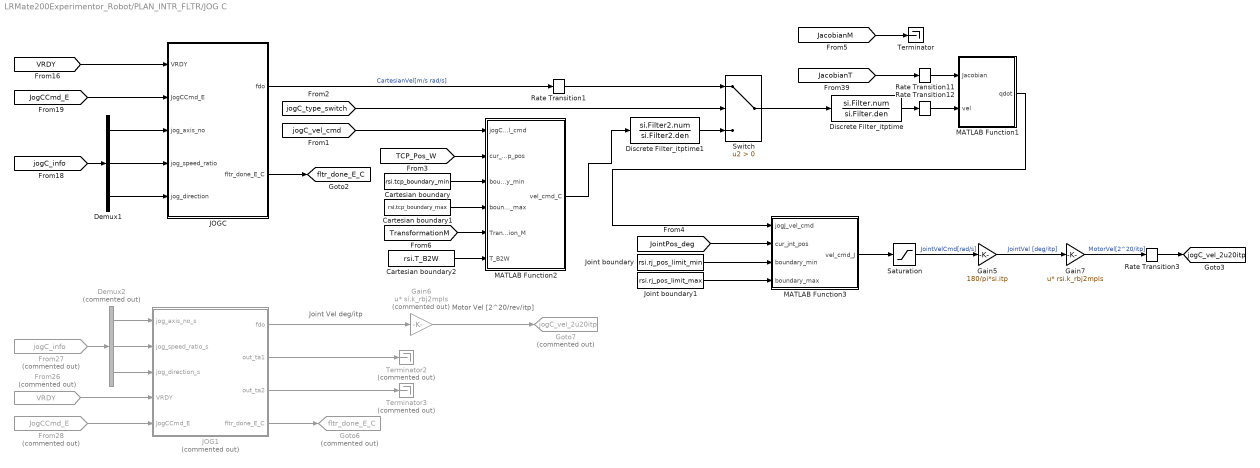
== system LRMate200Experimentor_Robot/PLAN_INTR_FLTR/JOG C ==
  note: Joint Vel deg/itp
  note: Motor Vel [2^20/rev/itp]
  Cartesian boundary : Constant  Value=rsi.tcp_boundary_min
  Cartesian boundary1 : Constant  Value=rsi.tcp_boundary_max
  Cartesian boundary2 : Constant  Value=rsi.T_B2W
  Demux1 : Demux  Outputs=3
  Demux2 : Demux  Commented=on  Outputs=3
  Discrete Filter_itptime : DiscreteFilter  Numerator=si.Filter.num  Denominator=si.Filter.den  SampleTime=si.tsv
  Discrete Filter_itptime1 : DiscreteFilter  Numerator=si.Filter2.num  Denominator=si.Filter2.den  SampleTime=si.tsv
  From26 : From  Commented=on  GotoTag=VRDY  TagVisibility=global
  From27 : From  Commented=on  GotoTag=jogC_info  TagVisibility=global
  From28 : From  Commented=on  GotoTag=JogCCmd_E  TagVisibility=global
  Gain5 : Gain  Gain=180/pi*si.itp
  Gain6 : Gain  Commented=on  Gain=si.k_rbj2mpls  Multiplication=Matrix(u*K)
  Gain7 : Gain  Gain=rsi.k_rbj2mpls  Multiplication=Matrix(u*K)
  Goto6 : Goto  Commented=on  GotoTag=fltr_done_E_C  TagVisibility=global
  Goto7 : Goto  Commented=on  GotoTag=jogC_vel_2u20itp  TagVisibility=global
  JOG1 : Stateflow chart  Commented=on  TreatAsAtomicUnit=on
  JOGC : Stateflow chart  TreatAsAtomicUnit=on
  Joint boundary : Constant  Value=rsi.rj_pos_limit_min
  Joint boundary1 : Constant  Value=rsi.rj_pos_limit_max
  MATLAB Function1 : MATLAB Function  TreatAsAtomicUnit=on
  MATLAB Function2 : MATLAB Function  TreatAsAtomicUnit=on
  MATLAB Function3 : MATLAB Function  TreatAsAtomicUnit=on
  Rate Transition{1,3,11..12} (4 alike) : RateTransition
  Saturation : Saturate  UpperLimit=30/180*pi*ones(1,6)  LowerLimit=-30/180*pi*ones(1,6)
  Switch : Switch  Criteria=u2 > Threshold
  Terminator : Terminator
  Terminator2 : Terminator  Commented=on
  Terminator3 : Terminator  Commented=on
  tag scope: fltr_done_E_C=global, jogC_vel_2u20itp=global
  wires:
  [VRDY] -> JOGC/1(VRDY)
  [jogC_info] -> Demux1/1
  [JogCCmd_E] -> JOGC/2(JogCCmd_E)
  JOGC/2(fltr_done_E_C) -> [fltr_done_E_C]
  JOGC/1(fdo) -> Rate Transition1/1  "CartesianVel[m/s rad/s]"
  Demux1/1 -> JOGC/3(jog_axis_no)
  Demux1/2 -> JOGC/4(jog_speed_ratio)
  Demux1/3 -> JOGC/5(jog_direction)
  JOG1/1(fdo) -> Gain6/1
  JOG1/2(out_ta1) -> Terminator2/1
  JOG1/3(out_ta2) -> Terminator3/1
  From28/1 -> JOG1/5(JogCCmd_E)
  From26/1 -> JOG1/4(VRDY)
  From27/1 -> Demux2/1
  Demux2/1 -> JOG1/1(jog_axis_no_s)
  Demux2/2 -> JOG1/2(jog_speed_ratio_s)
  Demux2/3 -> JOG1/3(jog_direction_s)
  JOG1/4(fltr_done_E_C) -> Goto6/1
  Gain6/1 -> Goto7/1
  Discrete Filter_itptime/1 -> Rate Transition12/1
  [JacobianT] -> Rate Transition11/1
  Rate Transition11/1 -> MATLAB Function1/1(Jacobian)
  Switch/1 -> Discrete Filter_itptime/1
  Rate Transition12/1 -> MATLAB Function1/2(vel)
  Saturation/1 -> Gain5/1  "JointVelCmd[rad/s]"
  Gain5/1 -> Gain7/1  "JointVel [deg/itp]"
  Gain7/1 -> Rate Transition3/1  "MotorVel[2^20/itp]"
  [jogC_type_switch] -> Switch/2
  [TCP_Pos_W] -> MATLAB Function2/2(cur_tcp_pos)
  [jogC_vel_cmd] -> MATLAB Function2/1(jogC_vel_cmd)
  Cartesian boundary/1 -> MATLAB Function2/3(boundary_min)
  MATLAB Function3/1(vel_cmd_J) -> Saturation/1
  MATLAB Function1/1(qdot) -> MATLAB Function3/1(jogJ_vel_cmd)
  [JointPos_deg] -> MATLAB Function3/2(cur_jnt_pos)
  Joint boundary/1 -> MATLAB Function3/3(boundary_min)
  Cartesian boundary1/1 -> MATLAB Function2/4(boundary_max)
  Joint boundary1/1 -> MATLAB Function3/4(boundary_max)
  MATLAB Function2/1(vel_cmd_C) -> Discrete Filter_itptime1/1
  Rate Transition3/1 -> [jogC_vel_2u20itp]
  Rate Transition1/1 -> Switch/1
  Discrete Filter_itptime1/1 -> Switch/3
  [JacobianM] -> Terminator/1
  [TransformationM] -> MATLAB Function2/5(Transformation_M)
  Cartesian boundary2/1 -> MATLAB Function2/6(T_B2W)

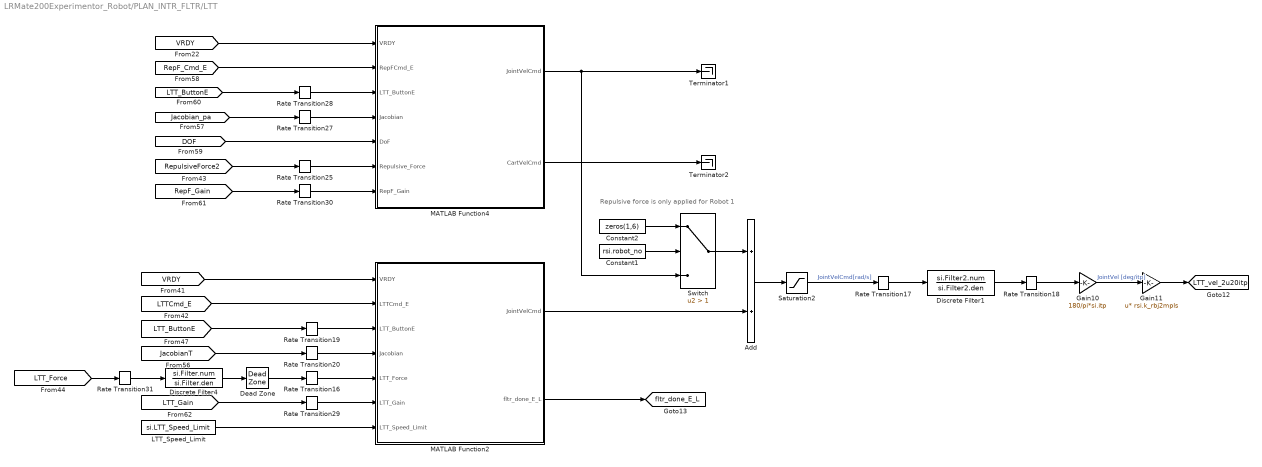
== system LRMate200Experimentor_Robot/PLAN_INTR_FLTR/LTT ==
  note: Repulsive force is only applied for Robot 1
  Add : Sum
  Constant1 : Constant  Value=rsi.robot_no
  Constant2 : Constant  Value=zeros(1,6)
  Dead Zone : DeadZone  LowerValue=-si.LTT_DeadZone  UpperValue=si.LTT_DeadZone  SaturateOnIntegerOverflow=on
  Discrete Filter1 : DiscreteFilter  Numerator=si.Filter2.num  Denominator=si.Filter2.den  SampleTime=si.tsv
  Discrete Filter4 : DiscreteFilter  Numerator=si.Filter.num  Denominator=si.Filter.den  SampleTime=si.tsv
  Gain10 : Gain  Gain=180/pi*si.itp
  Gain11 : Gain  Gain=rsi.k_rbj2mpls  Multiplication=Matrix(u*K)
  LTT_Speed_Limit : Constant  Value=si.LTT_Speed_Limit
  MATLAB Function2 : MATLAB Function  TreatAsAtomicUnit=on
  MATLAB Function4 : MATLAB Function  TreatAsAtomicUnit=on
  Rate Transition{16..20,25,27..31} (11 alike) : RateTransition
  Saturation2 : Saturate  UpperLimit=30/180*pi*ones(1,6)  LowerLimit=-30/180*pi*ones(1,6)
  Switch : Switch  Criteria=u2 > Threshold  Threshold=1
  Terminator1 : Terminator
  Terminator2 : Terminator
  tag scope: LTT_vel_2u20itp=global, fltr_done_E_L=global
  wires:
  [LTTCmd_E] -> MATLAB Function2/2(LTTCmd_E)
  Saturation2/1 -> Rate Transition17/1  "JointVelCmd[rad/s]"
  Discrete Filter1/1 -> Rate Transition18/1
  MATLAB Function2/2(fltr_done_E_L) -> [fltr_done_E_L]
  Rate Transition20/1 -> MATLAB Function2/4(Jacobian)
  Rate Transition16/1 -> MATLAB Function2/5(LTT_Force)
  Rate Transition17/1 -> Discrete Filter1/1
  Rate Transition18/1 -> Gain10/1
  [VRDY] -> MATLAB Function2/1(VRDY)
  Gain10/1 -> Gain11/1  "JointVel [deg/itp]"
  Gain11/1 -> [LTT_vel_2u20itp]
  Rate Transition19/1 -> MATLAB Function2/3(LTT_ButtonE)
  [LTT_ButtonE] -> Rate Transition19/1
  [JacobianT] -> Rate Transition20/1
  [VRDY] -> MATLAB Function4/1(VRDY)
  [RepulsiveForce2] -> Rate Transition25/1
  Rate Transition25/1 -> MATLAB Function4/6(Repulsive_Force)
  Rate Transition27/1 -> MATLAB Function4/4(Jacobian)
  [Jacobian_pa] -> Rate Transition27/1
  [RepF_Cmd_E] -> MATLAB Function4/2(RepFCmd_E)
  [DOF] -> MATLAB Function4/5(DoF)
  Rate Transition28/1 -> MATLAB Function4/3(LTT_ButtonE)
  [LTT_ButtonE] -> Rate Transition28/1
  [RepF_Gain] -> Rate Transition30/1
  [LTT_Gain] -> Rate Transition29/1
  MATLAB Function4/2(CartVelCmd) -> Terminator2/1
  Rate Transition29/1 -> MATLAB Function2/6(LTT_Gain)
  Rate Transition30/1 -> MATLAB Function4/7(RepF_Gain)
  Discrete Filter4/1 -> Dead Zone/1
  Rate Transition31/1 -> Discrete Filter4/1
  [LTT_Force] -> Rate Transition31/1
  Add/1 -> Saturation2/1
  MATLAB Function2/1(JointVelCmd) -> Add/2
  MATLAB Function4/1(JointVelCmd) -> Terminator1/1, Switch/3
  Constant1/1 -> Switch/2
  Constant2/1 -> Switch/1
  Switch/1 -> Add/1
  LTT_Speed_Limit/1 -> MATLAB Function2/7(LTT_Speed_Limit)
  Dead Zone/1 -> Rate Transition16/1

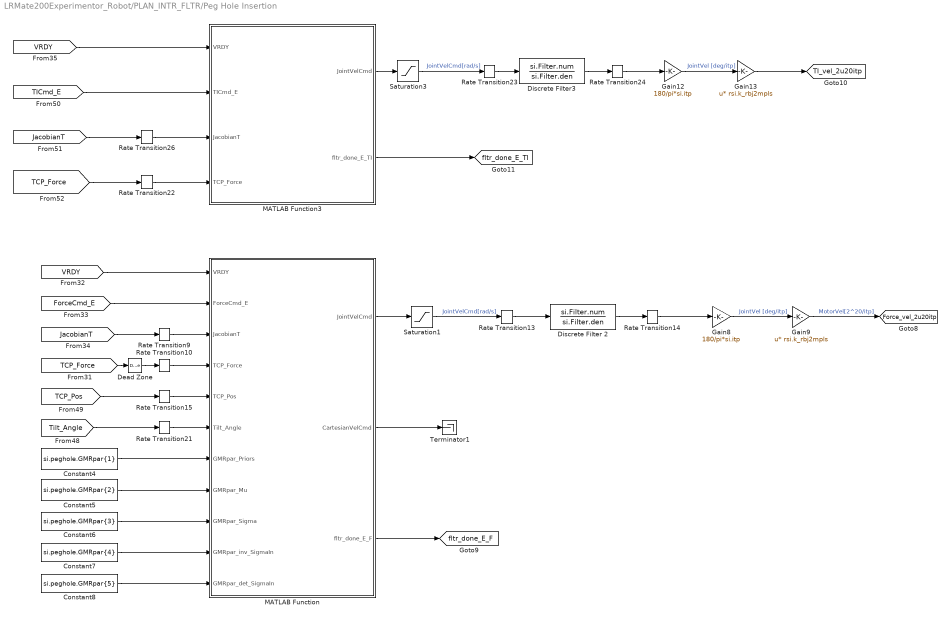
== system LRMate200Experimentor_Robot/PLAN_INTR_FLTR/Peg Hole Insertion ==
  Constant4 : Constant  Value=si.peghole.GMRpar{1}
  Constant5 : Constant  Value=si.peghole.GMRpar{2}
  Constant6 : Constant  Value=si.peghole.GMRpar{3}
  Constant7 : Constant  Value=si.peghole.GMRpar{4}
  Constant8 : Constant  Value=si.peghole.GMRpar{5}
  Dead Zone : DeadZone  LowerValue=[-0.5, -0.5, -0.5, -0.01 ,-0.01 , -0.01]  UpperValue=[0.5, 0.5, 0.5, 0.01 ,0.01 , 0.01]  SaturateOnIntegerOverflow=on
  Discrete Filter 2 : DiscreteFilter  Numerator=si.Filter.num  Denominator=si.Filter.den  SampleTime=si.tsv
  Discrete Filter3 : DiscreteFilter  Numerator=si.Filter.num  Denominator=si.Filter.den  SampleTime=si.tsv
  Gain12 : Gain  Gain=180/pi*si.itp
  Gain13 : Gain  Gain=rsi.k_rbj2mpls  Multiplication=Matrix(u*K)
  Gain8 : Gain  Gain=180/pi*si.itp
  Gain9 : Gain  Gain=rsi.k_rbj2mpls  Multiplication=Matrix(u*K)
  MATLAB Function : MATLAB Function  TreatAsAtomicUnit=on
  MATLAB Function3 : MATLAB Function  TreatAsAtomicUnit=on
  Rate Transition{9..10,13..15,21..24,26} (10 alike) : RateTransition
  Saturation1 : Saturate  UpperLimit=20/180*pi*ones(1,6)  LowerLimit=-20/180*pi*ones(1,6)
  Saturation3 : Saturate  UpperLimit=30/180*pi*ones(1,6)  LowerLimit=-30/180*pi*ones(1,6)
  Terminator1 : Terminator
  tag scope: Force_vel_2u20itp=global, TI_vel_2u20itp=global, fltr_done_E_F=global, fltr_done_E_TI=global
  wires:
  [TICmd_E] -> MATLAB Function3/2(TICmd_E)
  [JacobianT] -> Rate Transition26/1
  MATLAB Function3/1(JointVelCmd) -> Saturation3/1
  Saturation3/1 -> Rate Transition23/1  "JointVelCmd[rad/s]"
  Discrete Filter3/1 -> Rate Transition24/1
  MATLAB Function3/2(fltr_done_E_TI) -> [fltr_done_E_TI]
  Rate Transition26/1 -> MATLAB Function3/3(JacobianT)
  Rate Transition22/1 -> MATLAB Function3/4(TCP_Force)
  Rate Transition23/1 -> Discrete Filter3/1
  Rate Transition24/1 -> Gain12/1
  [VRDY] -> MATLAB Function3/1(VRDY)
  Gain12/1 -> Gain13/1  "JointVel [deg/itp]"
  Gain13/1 -> [TI_vel_2u20itp]
  [TCP_Force] -> Rate Transition22/1
  [ForceCmd_E] -> MATLAB Function/2(ForceCmd_E)
  [JacobianT] -> Rate Transition9/1
  [TCP_Force] -> Dead Zone/1
  MATLAB Function/1(JointVelCmd) -> Saturation1/1
  Saturation1/1 -> Rate Transition13/1  "JointVelCmd[rad/s]"
  Discrete Filter 2/1 -> Rate Transition14/1
  MATLAB Function/3(fltr_done_E_F) -> [fltr_done_E_F]
  Rate Transition9/1 -> MATLAB Function/3(JacobianT)
  Rate Transition10/1 -> MATLAB Function/4(TCP_Force)
  Rate Transition13/1 -> Discrete Filter 2/1
  [TCP_Pos] -> Rate Transition15/1
  Rate Transition15/1 -> MATLAB Function/5(TCP_Pos)
  Dead Zone/1 -> Rate Transition10/1
  [VRDY] -> MATLAB Function/1(VRDY)
  Constant4/1 -> MATLAB Function/7(GMRpar_Priors)
  Constant5/1 -> MATLAB Function/8(GMRpar_Mu)
  Constant6/1 -> MATLAB Function/9(GMRpar_Sigma)
  Constant7/1 -> MATLAB Function/10(GMRpar_inv_SigmaIn)
  Constant8/1 -> MATLAB Function/11(GMRpar_det_SigmaIn)
  MATLAB Function/2(CartesianVelCmd) -> Terminator1/1
  Rate Transition14/1 -> Gain8/1
  Gain8/1 -> Gain9/1  "JointVel [deg/itp]"
  Gain9/1 -> [Force_vel_2u20itp]  "MotorVel[2^20/itp]"
  [Tilt_Angle] -> Rate Transition21/1
  Rate Transition21/1 -> MATLAB Function/6(Tilt_Angle)

== system LRMate200Experimentor_Robot/Device Control/Gripper Input/SwSrc1 ==
  S0 : Constant  Value=0
  S1 : Constant
  ST1 : Outport
  ST0 : Outport  Port=2
  wires:
  S0/1 -> ST0/1
  S1/1 -> ST1/1

== system LRMate200Experimentor_Robot/Device Control/Gripper Input/SwSrc2 ==
  S0 : Constant  Value=0
  S1 : Constant
  ST1 : Outport
  ST0 : Outport  Port=2
  wires:
  S0/1 -> ST0/1
  S1/1 -> ST1/1

== system LRMate200Experimentor_Robot/Device Control/Gripper Input/SwSrc3 ==
  S0 : Constant  Value=0
  S1 : Constant
  ST1 : Outport
  ST0 : Outport  Port=2
  wires:
  S0/1 -> ST0/1
  S1/1 -> ST1/1

== system LRMate200Experimentor_Robot/Device Control/Gripper Input/SwSrc4 ==
  S0 : Constant  Value=0
  S1 : Constant
  ST1 : Outport
  ST0 : Outport  Port=2
  wires:
  S0/1 -> ST0/1
  S1/1 -> ST1/1

== system LRMate200Experimentor_Robot/Device Control/Gripper Input/SwSrc8 ==
  S0 : Constant  Value=0
  S1 : Constant
  ST1 : Outport
  ST0 : Outport  Port=2
  wires:
  S0/1 -> ST0/1
  S1/1 -> ST1/1

== system LRMate200Experimentor_Robot/Device Control/Gripper Input/Vector 2 Bus ==
  In1 : Inport
  Bus Creator : BusCreator  Inputs=6
  Demux : Demux  Outputs=6
  Rate Transition : RateTransition  OutPortSampleTime=si.timeGripperInputHold
  Out1 : Outport
  wires:
  Bus Creator/1 -> Out1/1
  In1/1 -> Rate Transition/1
  Demux/1 -> Bus Creator/1  "GPR_MODE"
  Demux/2 -> Bus Creator/2  "SETUP"
  Demux/3 -> Bus Creator/3  "HOLD"
  Demux/4 -> Bus Creator/4  "DRIVE"
  Demux/6 -> Bus Creator/6  "SVON"
  Demux/5 -> Bus Creator/5  "RESET"
  Rate Transition/1 -> Demux/1

== system LRMate200Experimentor_Robot/Measurement/System State/Subsystem ==
  In1 : Inport
  Bitwise Operator : simulink/Logic and Bit Operations/Bitwise Operator  logicop=AND  UseBitMask=on  BitMask=bin2dec('100000000')  BitMaskRealWorld=Stored Integer
  Demux2 : Demux  Outputs=6
  Gain3 : Gain  Gain=1/256  OutDataTypeStr=uint16
  Logical Operator : Logic  Inputs=6  AllPortsSameDT=off  OutDataTypeStr=boolean
  Rate5 : RateTransition  OutPortSampleTime=si.itp
  S1 : Constant  OutDataTypeStr=boolean
  Switch CurPos Run : ManualSwitch
  Out1 : Outport
  wires:
  Bitwise Operator/1 -> Gain3/1
  Gain3/1 -> Demux2/1
  Demux2/1 -> Logical Operator/1
  Demux2/2 -> Logical Operator/2
  Demux2/3 -> Logical Operator/3
  Demux2/4 -> Logical Operator/4
  Demux2/5 -> Logical Operator/5
  Demux2/6 -> Logical Operator/6
  Logical Operator/1 -> Switch CurPos Run/1
  S1/1 -> Switch CurPos Run/2
  Switch CurPos Run/1 -> Rate5/1
  Rate5/1 -> Out1/1
  In1/1 -> Bitwise Operator/1

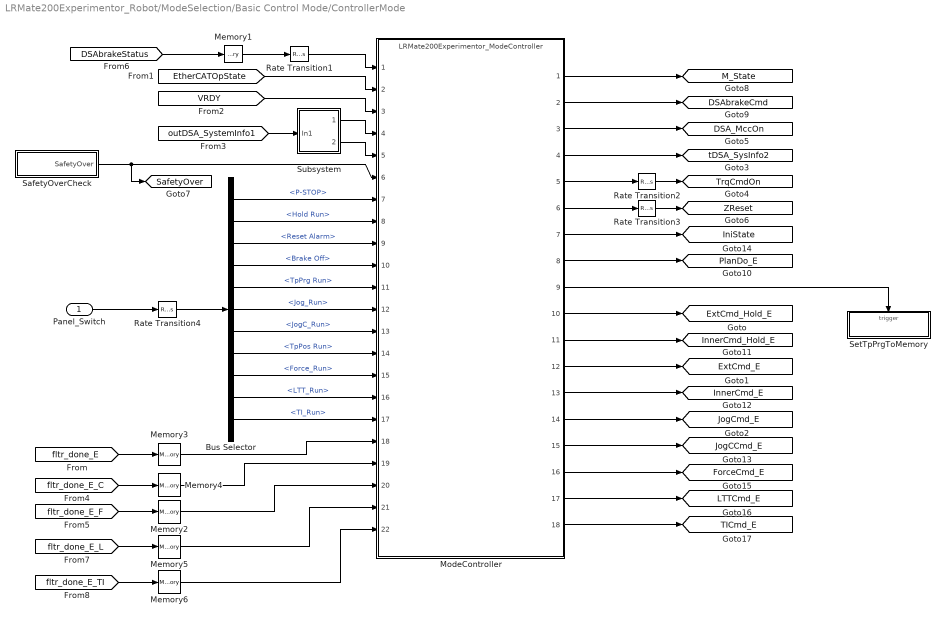
== system LRMate200Experimentor_Robot/ModeSelection/Basic Control Mode/ControllerMode ==
  Panel_Switch : Inport
  Bus Selector : BusSelector  OutputSignals=P-STOP,Hold Run,Reset Alarm,Brake Off,TpPrg Run,Jog_Run,JogC_Run,TpPos Run,Force_Run,LTT_Run,TI_Run
  Memory{1..6} (6 alike) : Memory  InheritSampleTime=on
  ModeController : ModelReference  ModelNameDialog=LRMate200Experimentor_ModeController.slx  SimulationMode=Normal  ModelReferenceVersion=1.75  CopyOfModelName=LRMate200Experimentor_ModeController.slx
  Rate Transition1 : RateTransition
  Rate Transition2 : RateTransition  OutPortSampleTime=si.tsv
  Rate Transition3 : RateTransition  OutPortSampleTime=si.tsv
  Rate Transition4 : RateTransition  OutPortSampleTime=si.itp
  SafetyOverCheck : Subsystem
  SetTpPrgToMemory : Subsystem  TreatAsAtomicUnit=on
  Subsystem : Subsystem
  tag scope: DSA_MccOn=global, DSAbrakeCmd=global, ExtCmd_E=global, ExtCmd_Hold_E=global, ForceCmd_E=global, IniState=global, InnerCmd_E=global, InnerCmd_Hold_E=global, JogCCmd_E=global, JogCmd_E=global, LTTCmd_E=global, M_State=global, PlanDo_E=global, SafetyOver=global, TICmd_E=global, TrqCmdOn=global, ZReset=global, tDSA_SysInfo2=global
  wires:
  [fltr_done_E] -> Memory3/1
  [DSAbrakeStatus] -> Memory1/1
  Memory1/1 -> Rate Transition1/1
  [outDSA_SystemInfo1] -> Subsystem/1(In1)
  SafetyOverCheck/1(SafetyOver) -> [SafetyOver], ModeController/6
  ModeController/2 -> [DSAbrakeCmd]
  ModeController/3 -> [DSA_MccOn]
  ModeController/4 -> [tDSA_SysInfo2]
  ModeController/1 -> [M_State]
  [fltr_done_E_C] -> Memory4/1
  Panel_Switch/1 -> Rate Transition4/1
  Rate Transition1/1 -> ModeController/1
  [EtherCATOpState] -> ModeController/2
  [VRDY] -> ModeController/3
  Subsystem/1(Out1) -> ModeController/4
  Subsystem/2(Out2) -> ModeController/5
  Bus Selector/3 -> ModeController/9  "<Reset Alarm>"
  Bus Selector/2 -> ModeController/8  "<Hold Run>"
  Bus Selector/1 -> ModeController/7  "<P-STOP>"
  Bus Selector/5 -> ModeController/11  "<TpPrg Run>"
  Bus Selector/8 -> ModeController/14  "<TpPos Run>"
  Bus Selector/6 -> ModeController/12  "<Jog_Run>"
  Bus Selector/7 -> ModeController/13  "<JogC_Run>"
  Bus Selector/4 -> ModeController/10  "<Brake Off>"
  [fltr_done_E_F] -> Memory2/1
  Bus Selector/9 -> ModeController/15  "<Force_Run>"
  Bus Selector/10 -> ModeController/16  "<LTT_Run>"
  [fltr_done_E_L] -> Memory5/1
  ModeController/5 -> Rate Transition2/1
  ModeController/6 -> Rate Transition3/1
  ModeController/7 -> [IniState]
  ModeController/8 -> [PlanDo_E]
  ModeController/9 -> SetTpPrgToMemory/Trigger
  ModeController/10 -> [ExtCmd_Hold_E]
  ModeController/11 -> [InnerCmd_Hold_E]
  ModeController/12 -> [ExtCmd_E]
  ModeController/13 -> [InnerCmd_E]
  ModeController/14 -> [JogCmd_E]
  ModeController/15 -> [JogCCmd_E]
  ModeController/16 -> [ForceCmd_E]
  ModeController/17 -> [LTTCmd_E]
  [fltr_done_E_TI] -> Memory6/1
  Bus Selector/11 -> ModeController/17  "<TI_Run>"
  Memory3/1 -> ModeController/18
  Memory4/1 -> ModeController/19
  Memory2/1 -> ModeController/20
  Memory5/1 -> ModeController/21
  Memory6/1 -> ModeController/22
  ModeController/18 -> [TICmd_E]
  Rate Transition2/1 -> [TrqCmdOn]
  Rate Transition3/1 -> [ZReset]
  Rate Transition4/1 -> Bus Selector/1

== system LRMate200Experimentor_Robot/ModeSelection/Basic Control Mode/SwSrc1 ==
  S0 : Constant  Value=0
  S1 : Constant
  ST1 : Outport
  ST0 : Outport  Port=2
  wires:
  S0/1 -> ST0/1
  S1/1 -> ST1/1

== system LRMate200Experimentor_Robot/ModeSelection/Basic Control Mode/SwSrc10 ==
  S0 : Constant  Value=0
  S1 : Constant
  ST1 : Outport
  ST0 : Outport  Port=2
  wires:
  S0/1 -> ST0/1
  S1/1 -> ST1/1

== system LRMate200Experimentor_Robot/ModeSelection/Basic Control Mode/SwSrc11 ==
  S0 : Constant  Value=0
  S1 : Constant
  ST1 : Outport
  ST0 : Outport  Port=2
  wires:
  S0/1 -> ST0/1
  S1/1 -> ST1/1

== system LRMate200Experimentor_Robot/ModeSelection/Basic Control Mode/SwSrc12 ==
  S0 : Constant  Value=0
  S1 : Constant
  ST1 : Outport
  ST0 : Outport  Port=2
  wires:
  S0/1 -> ST0/1
  S1/1 -> ST1/1

== system LRMate200Experimentor_Robot/ModeSelection/Basic Control Mode/SwSrc14 ==
  S0 : Constant  Value=0
  S1 : Constant
  ST1 : Outport
  ST0 : Outport  Port=2
  wires:
  S0/1 -> ST0/1
  S1/1 -> ST1/1

== system LRMate200Experimentor_Robot/ModeSelection/Basic Control Mode/SwSrc2 ==
  S0 : Constant  Value=0
  S1 : Constant
  ST1 : Outport
  ST0 : Outport  Port=2
  wires:
  S0/1 -> ST0/1
  S1/1 -> ST1/1

== system LRMate200Experimentor_Robot/ModeSelection/Basic Control Mode/SwSrc3 ==
  S0 : Constant  Value=0
  S1 : Constant
  ST1 : Outport
  ST0 : Outport  Port=2
  wires:
  S0/1 -> ST0/1
  S1/1 -> ST1/1

== system LRMate200Experimentor_Robot/ModeSelection/Basic Control Mode/SwSrc4 ==
  S0 : Constant  Value=0
  S1 : Constant
  ST1 : Outport
  ST0 : Outport  Port=2
  wires:
  S0/1 -> ST0/1
  S1/1 -> ST1/1

== system LRMate200Experimentor_Robot/ModeSelection/Basic Control Mode/SwSrc6 ==
  S0 : Constant  Value=0
  S1 : Constant
  ST1 : Outport
  ST0 : Outport  Port=2
  wires:
  S0/1 -> ST0/1
  S1/1 -> ST1/1

== system LRMate200Experimentor_Robot/ModeSelection/Basic Control Mode/SwSrc7 ==
  S0 : Constant  Value=0
  S1 : Constant
  ST1 : Outport
  ST0 : Outport  Port=2
  wires:
  S0/1 -> ST0/1
  S1/1 -> ST1/1

== system LRMate200Experimentor_Robot/ModeSelection/Basic Control Mode/SwSrc8 ==
  S0 : Constant  Value=0
  S1 : Constant
  ST1 : Outport
  ST0 : Outport  Port=2
  wires:
  S0/1 -> ST0/1
  S1/1 -> ST1/1
